simulink model "modelo_stateflow"  (R2021a)
settings: Solver=VariableStepAuto  StartTime=0.0  StopTime=10.0  RelTol=1e-3
settings Model: Creator=Mariano  LastModifiedBy=Mariano

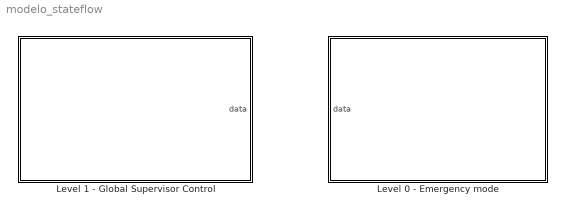
== system modelo_stateflow ==
  Level 0 - Emergency mode : Stateflow chart  TreatAsAtomicUnit=on
  Level 1 - Global Supervisor Control : Stateflow chart  TreatAsAtomicUnit=on

== stateflow chart modelo_stateflow/Level 0 - Emergency mode ==
  data: data input

== stateflow chart modelo_stateflow/Level 1 - Global Supervisor Control ==
  state MANUAL
    entry: move_t=0, move_h=0;
    state ALL_MANUAL
      state HOISTING [parallel]
        entry: limits_h=0;
        settings: executionOrder=1
        state MOVE
          during:
          dy=VYh*move_h;
        state STOP
          entry:
          dy=0;
        (default) -> MANUAL.ALL_MANUAL.HOISTING.MOVE
        MANUAL.ALL_MANUAL.HOISTING.STOP -> MANUAL.ALL_MANUAL.HOISTING.MOVE : [move_h~=0 || limits_h==0;]
        MANUAL.ALL_MANUAL.HOISTING.MOVE -> MANUAL.ALL_MANUAL.HOISTING.STOP : [move_h==0 || limits_h==1;]
      state TROLLEY [parallel]
        entry: limits_t=0;
        settings: executionOrder=2
        state STOP
          entry:
          dx=0;
        state MOVE
          during:
          dx=VXt*move_t;
        (default) -> MANUAL.ALL_MANUAL.TROLLEY.MOVE
        MANUAL.ALL_MANUAL.TROLLEY.STOP -> MANUAL.ALL_MANUAL.TROLLEY.MOVE : [move_t~=0 || limits_t==0;]
        MANUAL.ALL_MANUAL.TROLLEY.MOVE -> MANUAL.ALL_MANUAL.TROLLEY.STOP : [move_t==0 || limits_t==1;]
    state HYBRID_MANUAL
      state HOISTING [parallel]
        entry: limits_h=0;
        settings: executionOrder=1
        state MOVE
          during:
          dy=VYh*move_h;
        state STOP
          entry:
          dy=0;
        (default) -> MANUAL.HYBRID_MANUAL.HOISTING.MOVE
        MANUAL.HYBRID_MANUAL.HOISTING.STOP -> MANUAL.HYBRID_MANUAL.HOISTING.MOVE : [move_h~=0 || limits_h==0;]
        MANUAL.HYBRID_MANUAL.HOISTING.MOVE -> MANUAL.HYBRID_MANUAL.HOISTING.STOP : [move_h==0 || limits_h==1;]
      state TROLLEY [parallel]
        entry: limits_t=0;
        settings: executionOrder=2
        state STOP
          entry:
          dx=0;
        state MOVE
          during:
          dx=VXt*move_t;
        (default) -> MANUAL.HYBRID_MANUAL.TROLLEY.MOVE
        MANUAL.HYBRID_MANUAL.TROLLEY.STOP -> MANUAL.HYBRID_MANUAL.TROLLEY.MOVE : [move_t~=0 || limits_t==0;]
        MANUAL.HYBRID_MANUAL.TROLLEY.MOVE -> MANUAL.HYBRID_MANUAL.TROLLEY.STOP : [move_t==0 || limits_t==1;]
    (default) -> ALL_MANUAL
    ALL_MANUAL -> HYBRID_MANUAL : [hybrid_mode == 1;]
    HYBRID_MANUAL -> ALL_MANUAL [order 1] : [hybrid_mode == 0]
  note: Descripción de ciclos:
      | -SIMPLE:
      | O se carga o se descarga, es decir: Si estoy cargando el barco, en el tramo muelle -> barco llevo un contenedor, pero vuelvo vacio. Es decir que el tramo barco -> muelle es sin ningun contenedor. Lo mismo sucederia si estoy descargando el barco: el tramo barco -> muelle es con un contenedor cargado, pero el tramo muelle -> barco es en vacio.
      | - DOBLE:
      | Se puede cargar y descargar en el mismo ciclo de trabajo. Es decir, que el tramo muelle -> barco es con un contenedor cargado, y el tramo barco -> muelle también. Por ende, se permite una carga intermedia antes de volver al muelle.
      |
      | ETAPAS DE LA TRAYECTORIA:
      | Cada stage se va aactivando dependiendo del punto de la trayectoria en el que se encuentra el barco
      | - STAGE 1 -> ground - el contenedor esta en tierra
      | - STAGE 2 -> el contenedor se encuentra en el aire (sobre muelle), en el punto de transicion manual a automatico.
      | - STAGE 3 -> el contenedor se enceuntra en el aire (sobre barco) ,en el punto de transicion automatico a manual.
      | - STAGE 4 -> el contenedor se encuentra en el barco.
  state AUTOMATIC
    entry: bot_cy=0;
    state INIT
    state DOUBLE_CYCLE
      state WAITING
      (default) -> AUTOMATIC.DOUBLE_CYCLE.WAITING
    state SINGLE_CYCLE
      entry: loading=2;
      state WAITING
      state LOADING
        state TO_SHIP
          during:
          dx = VXt*0.1;
          dy = VYh*0.1;
        state INIT
        state TO_DOCK
          during:
          dx = VXt*0.5;
          dy = VYh*0.5;
        AUTOMATIC.SINGLE_CYCLE.LOADING.INIT -> AUTOMATIC.SINGLE_CYCLE.LOADING.TO_SHIP [order 1] : [current_stage == 2 && prev_stage == 1;]
        (default) -> AUTOMATIC.SINGLE_CYCLE.LOADING.INIT
        AUTOMATIC.SINGLE_CYCLE.LOADING.INIT -> AUTOMATIC.SINGLE_CYCLE.LOADING.TO_DOCK [order 2] : [current_stage == 3 && prev_stage == 4;]
      state UNLOADING
        state TO_SHIP
          during:
          dx = VXt*0.5;
          dy = VYh*0.5;
        state INIT
        state TO_DOCK
          during:
          dx = VXt*0.1;
          dy = VYh*0.1;
        AUTOMATIC.SINGLE_CYCLE.UNLOADING.INIT -> AUTOMATIC.SINGLE_CYCLE.UNLOADING.TO_SHIP [order 2] : [current_stage == 2 && prev_stage == 1;]
        (default) -> AUTOMATIC.SINGLE_CYCLE.UNLOADING.INIT
        AUTOMATIC.SINGLE_CYCLE.UNLOADING.INIT -> AUTOMATIC.SINGLE_CYCLE.UNLOADING.TO_DOCK [order 1] : [current_stage == 3 && prev_stage == 4]
      (default) -> AUTOMATIC.SINGLE_CYCLE.WAITING
      AUTOMATIC.SINGLE_CYCLE.WAITING -> LOADING [order 1] : [loading == 1 && unloading ==0;]
      AUTOMATIC.SINGLE_CYCLE.WAITING -> UNLOADING [order 2] : [loading == 0 && unloading == 1]
    (default) -> AUTOMATIC.INIT
    AUTOMATIC.INIT -> SINGLE_CYCLE [order 2] : [single_cycle==1;]
    AUTOMATIC.INIT -> DOUBLE_CYCLE [order 1] : [double_cycle==1;]
  note: Descripcion variables:
      | CARRO (TROLLEY):
      | - move_t -> (variable,int) boton para mover el carro en x.
      | - dx -> (variable,double) velocidad actual del carro (variable)
      | - VXt -> velocidad máxima del carro (es una constante, que al multiplicarla por bot_t modifica el valor de la velocidad real de carro.)
      | - limits_t -> (variable,bool) la variable cambia al valor 1 si se alcanzan los limites de movimiento del carro.
      |
      | IZAJE (HOISTING):
      | - move_h ->(variable,int) boton para izar la carga.
      | - dy -> (variable,double) velocidad actual del izaje.
      | - VYh -> (constante) velocidad máxima que puede alcanzar el izaje.
      | - limits_h -> (variable,bool) la variable cambia al valor 1 si se alcanzan los limites de movimiento del izaje.
      |
      | Descripcion de bloques:
      | - ALL_MANUAL:
      | Es el modo manual por defecto, el operario puede manejar el trolley y el hoisting con 2 botones. El boton move_t se encarga de mover el trolley y el boton move_h de izar la carga.
      | - HYRBID_MANUAL:
      | Es el modo manual que esta presente en los ciclos simple o doble. Es decir, esta intercalado con el modo automático
  (default) -> MANUAL
  HYBRID_MANUAL -> AUTOMATIC [order 2] : [(current_stage ==  2 && prev_stage == 1) && auto_mode == 1;]
  HYBRID_MANUAL -> AUTOMATIC [order 3] : [current_stage == 3 && prev_stage == 4 && auto_mode == 1]
  AUTOMATIC.SINGLE_CYCLE.LOADING.TO_SHIP -> HYBRID_MANUAL : [current_stage == 3 && prev_stage == 2;]
  AUTOMATIC.SINGLE_CYCLE.LOADING.TO_DOCK -> HYBRID_MANUAL : [current_stage == 2 && prev_stage == 3]
  AUTOMATIC.SINGLE_CYCLE.UNLOADING.TO_SHIP -> HYBRID_MANUAL : [current_stage == 3 && prev_stage == 2;]
  AUTOMATIC.SINGLE_CYCLE.UNLOADING.TO_DOCK -> HYBRID_MANUAL : [current_stage == 2 && prev_stage == 3;]
  data: data output
